simulink model "Yaw_Simulation"  (R2022b)
settings: Solver=VariableStepAuto  StartTime=0.0  StopTime=5  RelTol=1e-3
values from neighbouring files (symbols this model uses):
  Kd_PitchRate_val = 18e6    (= 18000000)    [Yaw_TF_Analysis.m]
  Ki_PitchRate_val = 9e6    (= 9000000)    [Yaw_TF_Analysis.m]
  Kp_PitchRate_val = 20e6    (= 20000000)    [Yaw_TF_Analysis.m]
  N_PitchRate_val = 10    [Yaw_TF_Analysis.m]
undefined symbols (not defined in the file or in its folder): Ts
libraries: slpidlib x1
settings Model: Creator=marcv  LastModifiedBy=marcv

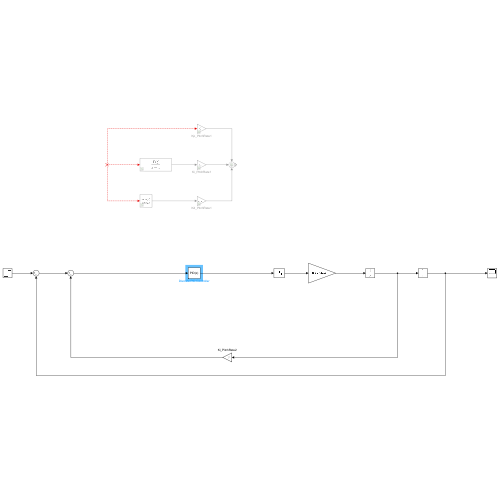
[thumbnail: Simulink's stored preview of the top-level diagram]
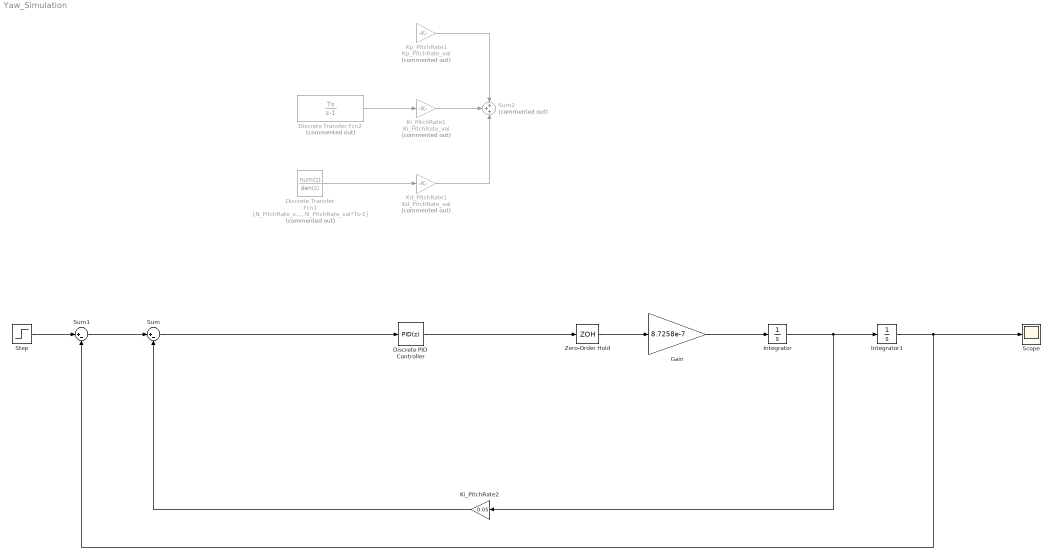
== system Yaw_Simulation ==
  Discrete Transfer Fcn1 : DiscreteTransferFcn  Commented=on  Numerator=[N_PitchRate_val, -N_PitchRate_val]  Denominator=[1, N_PitchRate_val*Ts-1]  SampleTime=Ts
  Discrete Transfer Fcn2 : DiscreteTransferFcn  Commented=on  Numerator=Ts  Denominator=[1,-1]  SampleTime=Ts
  Discrete PID Controller : slpidlib/PID Controller  Controller=PID  Form=Parallel  TimeDomain=Discrete-time  UseExternalTs=off  SampleTime=-1  IntegratorMethod=Forward Euler  FilterMethod=Forward Euler  ControllerParametersSource=internal  P=19725613.0665696  I=8798493.62968835  UseKiTs=off  D=10566487.4559227  N=32.518698085206  UseFilter=on  TunerSelectOption=Transfer Function Based (PID Tuner App)  InitialConditionSource=internal  InitialConditionForIntegrator=0  InitialConditionForFilter=0  DifferentiatorICPrevScaledInput=0  ExternalReset=none  TrackingMode=off  Kt=1  LimitOutput=off  SatLimitsSource=internal  UpperSaturationLimit=inf  LowerSaturationLimit=-inf  LinearizeAsGain=off  AntiWindupMode=none  Kb=1  LimitIntegrator=off  UpperIntegratorSaturationLimit=inf  LowerIntegratorSaturationLimit=-inf  POutMin=[]  POutMax=[]  IOutMin=[]  IOutMax=[]  DOutMin=[]  DOutMax=[]  NOutMin=[]  NOutMax=[]  SumOutMin=[]  SumOutMax=[]  SaturationOutMin=[]  SaturationOutMax=[]  PParamMin=[]  PParamMax=[]  IParamMin=[]  IParamMax=[]  DParamMin=[]  DParamMax=[]  NParamMin=[]  NParamMax=[]  KbParamMin=[]  KbParamMax=[]  KtParamMin=[]  KtParamMax=[]  KbOutMin=[]  KbOutMax=[]  KtOutMin=[]  KtOutMax=[]  IntegratorOutMin=[]  IntegratorOutMax=[]  FilterOutMin=[]  FilterOutMax=[]  SumI1OutMin=[]  SumI1OutMax=[]  SumI2OutMin=[]  SumI2OutMax=[]  SumI3OutMin=[]  SumI3OutMax=[]  SumI4OutMin=[]  SumI4OutMax=[]  SumDOutMin=[]  SumDOutMax=[]  DifferentiatorOutMin=[]  DifferentiatorOutMax=[]  FilterDiffOutCoefMin=[]  FilterDiffOutCoefMax=[]  ReciprocalOutMin=[]  ReciprocalOutMax=[]  SumDenOutMin=[]  SumDenOutMax=[]  SumNumOutMin=[]  SumNumOutMax=[]  DivideOutMin=[]  DivideOutMax=[]  UdiffTsProdOutMin=[]  UdiffTsProdOutMax=[]  NTsProdOutMin=[]  NTsProdOutMax=[]  UintegralTsProdOutMin=[]  UintegralTsProdOutMax=[]  UngainTsProdOutMin=[]  UngainTsProdOutMax=[]  ClampingZeroOutDataTypeStr=Inherit: Inherit via back propagation  ClampingZeroOutMin=[]  ClampingZeroOutMax=[]  FilterDenConstantOutDataTypeStr=Inherit: Inherit via back propagation  FilterDenConstantOutMin=[]  FilterDenConstantOutMax=[]  PCopyOutDataTypeStr=Inherit: Inherit via back propagation  PCopyOutMin=[]  PCopyOutMax=[]  NCopyOutDataTypeStr=Inherit: Inherit via back propagation  NCopyOutMin=[]  NCopyOutMax=[]  IntegratorContinuousStateAttributes=''  IntegratorStateMustResolveToSignalObject=off  IntegratorRTWStateStorageClass=Auto  FilterContinuousStateAttributes=''  FilterStateMustResolveToSignalObject=off  FilterRTWStateStorageClass=Auto  ParallelPVariant=InternalParameters  IdealPVariant=Disabled  IVariant=InternalParameters  DVariant=InternalParameters  IntegratorVariant=Discrete  SatVariant=Disabled  AWVariant=Passthrough  PCopyVariant=Disabled  TRVariant=Disabled  FdbkBlocksVariant=Forward  IdealPFdbkVariant=Disabled  SatFdbkVariant=Disabled  DerivativeFilterVariant=ForwardEulerFilter  NVariant=InternalParameters  NCopyVariant=Disabled  FilterICVariant=InternalICsFilter  IntegratorICVariant=InternalICs  ExternalResetVariant=Disabled  TRSumVariant=Passthrough  SumFdbkVariant=Disabled  SumVariant=Sum_PID  TsampFilterVariant=InternalTs  TsampNgainVariant=Passthrough  TsampIntegralVariant=Passthrough  ExternalSaturationOutDataTypeStr=Inherit: Same as second input
      settings: LibrarySourceBlock=simulink/Discrete/Discrete PID Controller
  Gain : Gain  Gain=8.7258e-7
  Integrator : Integrator
  Integrator1 : Integrator
  Kd_PitchRate1 : Gain  Commented=on  Gain=Kd_PitchRate_val
  Ki_PitchRate1 : Gain  Commented=on  Gain=Ki_PitchRate_val
  Ki_PitchRate2 : Gain  Gain=0.05
  Kp_PitchRate1 : Gain  Commented=on  Gain=Kp_PitchRate_val
  Scope : Scope
  Step : Step  SampleTime=0
  Sum : Sum  Inputs=|+-
  Sum1 : Sum  Inputs=|+-
  Sum2 : Sum  Commented=on  Inputs=+++
  Zero-Order Hold : ZeroOrderHold  SampleTime=0.01
  wires:
  Sum1/1 -> Sum/1
  Discrete PID Controller/1 -> Zero-Order Hold/1
  Zero-Order Hold/1 -> Gain/1
  Gain/1 -> Integrator/1
  Integrator/1 -> Ki_PitchRate2/1, Integrator1/1
  Integrator1/1 -> Scope/1, Sum1/2
  Step/1 -> Sum1/1
  Ki_PitchRate2/1 -> Sum/2
  Sum/1 -> Discrete PID Controller/1
  ? -> Discrete Transfer Fcn2/1
  Ki_PitchRate1/1 -> Sum2/2
  Kp_PitchRate1/1 -> Sum2/1
  Kd_PitchRate1/1 -> Sum2/3
  ? -> Kp_PitchRate1/1
  Discrete Transfer Fcn1/1 -> Kd_PitchRate1/1
  ? -> Discrete Transfer Fcn1/1
  Discrete Transfer Fcn2/1 -> Ki_PitchRate1/1
